simulink model "Model_IPS7"  (R2016a)
settings: Solver=FixedStepAuto  StartTime=0  StopTime=2  FixedStep=1e-5
InitFcn:
  | parametriAM
values from neighbouring files (symbols this model uses):
  filtkonst = 1.3    [parametriAM.m]
  Imrn = 7.4    [parametriAM.m]
  In = 12.7    [parametriAM.m]
  Ismax = In*sqrt(2)    [parametriAM.m]
  J = 0.019    [parametriAM.m]
  Ki_Imr = 1000    [parametriAM.m]
  Ki_tok = 5.0    (= 5)    [parametriAM.m]
  Ki_wr = 1000    [parametriAM.m]
  Kp_Imr = 100    [parametriAM.m]
  Kp_tok = 0.05    [parametriAM.m]
  Kp_wr = 50    [parametriAM.m]
  Lm = 0.0493    [parametriAM.m]
  Lr = 0.05315    [parametriAM.m]
  Ls = 0.05315    [parametriAM.m]
  Lst = sigma*Ls    (= 0.00742111947319)    [parametriAM.m]
  pp = 3    [parametriAM.m]
  Rs = 0.594    [parametriAM.m]
  sigma = 1 - 1/((1+sigmaR)*(1+sigmaS))    (= 0.13962595434)    [parametriAM.m]
  Tr = Lr/Rr    (= 0.0771407837446)    [parametriAM.m]
  Udc = Un*sqrt(2)    [parametriAM.m]
  wb_upper_limit_field_weaking = sqrt((Ls^2+Lst^2)/(2*Lst^2*Ls^2))*Usmax/Ismax    [parametriAM.m]
  wdod = 2000*2*pi/60    (= 209.439510239)    [parametriAM.m]
libraries: simulink x18
(part 1 of 2)
settings Model: Creator=Vaje  LastModifiedBy=Mitja1

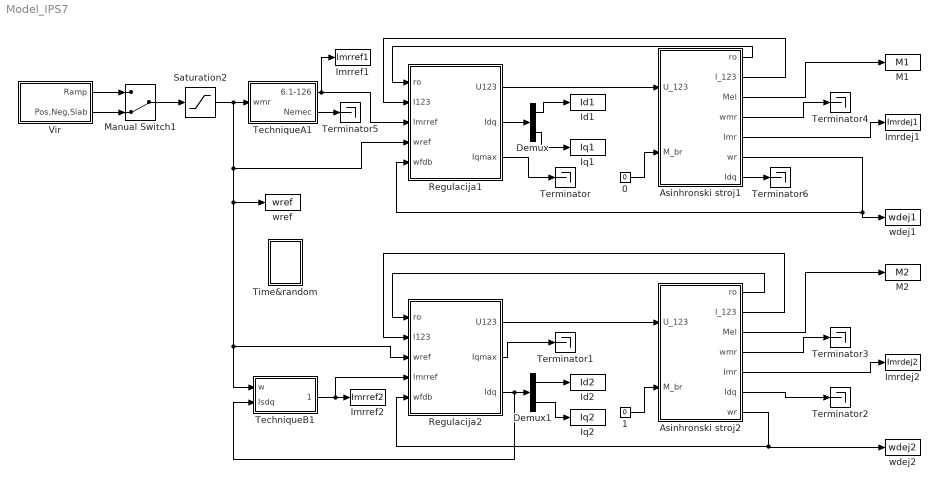
== system Model_IPS7 ==
  0 : Constant  Value=0
  1 : Constant  Value=0
  Asinhronski stroj1 : Subsystem  InitFcn=parametriAM
  Asinhronski stroj2 : Subsystem  InitFcn=parametriAM
  Demux : Demux  Outputs=2
  Demux1 : Demux  Outputs=2
  Id1 : ToWorkspace  VariableName=Id1  SampleTime=-1
      settings: Decimation=3  Save2DSignal=2-D array (concatenate along first dimension)
  Id2 : ToWorkspace  VariableName=Id2  SampleTime=-1
      settings: Decimation=3  Save2DSignal=2-D array (concatenate along first dimension)
  Imrdej1 : ToWorkspace  VariableName=Imrdej1  SampleTime=-1
      settings: Decimation=3  Save2DSignal=2-D array (concatenate along first dimension)
  Imrdej2 : ToWorkspace  VariableName=Imrdej2  SampleTime=-1
      settings: Decimation=3  Save2DSignal=2-D array (concatenate along first dimension)
  Imrref1 : ToWorkspace  VariableName=Imrref1  SampleTime=-1
      settings: Decimation=3  Save2DSignal=2-D array (concatenate along first dimension)
  Imrref2 : ToWorkspace  VariableName=Imrref2  SampleTime=-1
      settings: Decimation=3  Save2DSignal=2-D array (concatenate along first dimension)
  Iq1 : ToWorkspace  VariableName=Iq1  SampleTime=-1
      settings: Decimation=3  Save2DSignal=2-D array (concatenate along first dimension)
  Iq2 : ToWorkspace  VariableName=Iq2  SampleTime=-1
      settings: Decimation=3  Save2DSignal=2-D array (concatenate along first dimension)
  M1 : ToWorkspace  VariableName=M1  SampleTime=-1
      settings: Decimation=3  Save2DSignal=2-D array (concatenate along first dimension)
  M2 : ToWorkspace  VariableName=M2  SampleTime=-1
      settings: Decimation=3  Save2DSignal=2-D array (concatenate along first dimension)
  Manual Switch1 : ManualSwitch  CurrentSetting=0
  Regulacija1 : Subsystem
  Regulacija2 : Subsystem
  Saturation2 : Saturate  UpperLimit=wb_upper_limit_field_weaking  LowerLimit=-wb_upper_limit_field_weaking
  TechniqueA1 : Subsystem
  TechniqueB1 : Subsystem
  Terminator{,1..6} (7 alike) : Terminator
  Time&random : Subsystem
  Vir : Subsystem
  wdej1 : ToWorkspace  VariableName=wdej1  SampleTime=-1
      settings: Decimation=3  Save2DSignal=2-D array (concatenate along first dimension)
  wdej2 : ToWorkspace  VariableName=wdej2  SampleTime=-1
      settings: Decimation=3  Save2DSignal=2-D array (concatenate along first dimension)
  wref : ToWorkspace  VariableName=wref  SampleTime=-1
      settings: Decimation=3  Save2DSignal=2-D array (concatenate along first dimension)
  wires:
  Vir/1(Ramp) -> Manual Switch1/1
  Vir/2(Pos,Neg,Slab) -> Manual Switch1/2
  TechniqueA1/1(6.1-126) -> Regulacija1/3(Imrref), Imrref1/1
  Asinhronski stroj1/1(ro) -> Regulacija1/1(ro)
  Asinhronski stroj1/2(I_123) -> Regulacija1/2(I123)
  Regulacija1/1(U123) -> Asinhronski stroj1/1(U_123)
  Asinhronski stroj1/6(wr) -> Regulacija1/5(wfdb), wdej1/1
  Manual Switch1/1 -> Saturation2/1
  Asinhronski stroj2/1(ro) -> Regulacija2/1(ro)
  Asinhronski stroj2/2(I_123) -> Regulacija2/2(I123)
  Regulacija2/1(U123) -> Asinhronski stroj2/1(U_123)
  Asinhronski stroj2/7(wr) -> Regulacija2/5(wfdb), wdej2/1
  Saturation2/1 -> Regulacija1/4(wref), Regulacija2/3(wref), TechniqueB1/1(w), wref/1, TechniqueA1/1(wmr)
  Regulacija2/3(Idq) -> TechniqueB1/2(Isdq), Demux1/1
  TechniqueB1/1(6.1-135) -> Regulacija2/4(Imrref), Imrref2/1
  Asinhronski stroj1/5(Imr) -> Imrdej1/1
  Asinhronski stroj2/5(Imr) -> Imrdej2/1
  Asinhronski stroj1/3(Mel) -> M1/1
  Asinhronski stroj2/3(Mel) -> M2/1
  Demux/2 -> Iq1/1
  Demux/1 -> Id1/1
  Demux1/1 -> Id2/1
  Demux1/2 -> Iq2/1
  Regulacija1/2(Idq) -> Demux/1
  Regulacija1/3(Iqmax) -> Terminator/1
  Regulacija2/2(Iqmax) -> Terminator1/1
  Asinhronski stroj2/6(Idq) -> Terminator2/1
  Asinhronski stroj2/4(wmr) -> Terminator3/1
  Asinhronski stroj1/4(wmr) -> Terminator4/1
  TechniqueA1/2(Nemec) -> Terminator5/1
  0/1 -> Asinhronski stroj1/2(M_br)
  1/1 -> Asinhronski stroj2/2(M_br)
  Asinhronski stroj1/7(Idq) -> Terminator6/1

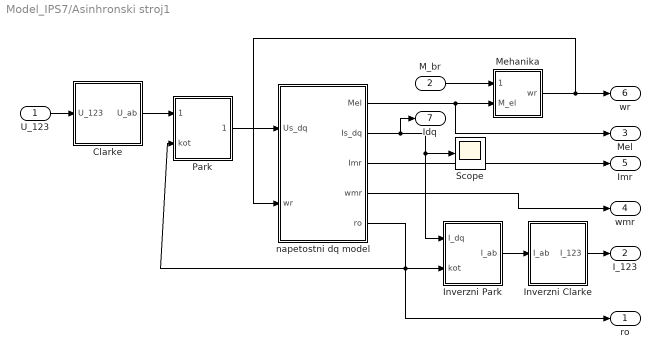
== system Model_IPS7/Asinhronski stroj1 ==
  U_123 : Inport
  M_br : Inport  Port=2
  Clarke : Subsystem
  Inverzni Clarke : Subsystem
  Inverzni Park : Subsystem
  Mehanika : Subsystem
  Park : Subsystem
  Scope : Scope
  napetostni dq model : Subsystem
  ro : Outport
  I_123 : Outport  Port=2
  Mel : Outport  Port=3
  wmr : Outport  Port=4
  Imr : Outport  Port=5
  wr : Outport  Port=6
  Idq : Outport  Port=7
  wires:
  Inverzni Park/1(I_ab) -> Inverzni Clarke/1(I_ab)
  Clarke/1(U_ab) -> Park/1(U_ab)
  Mehanika/1(wr) -> napetostni dq model/2(wr), wr/1
  M_br/1 -> Mehanika/1(M_br)
  napetostni dq model/1(Mel) -> Mel/1, Mehanika/2(M_el)
  Inverzni Clarke/1(I_123) -> I_123/1
  napetostni dq model/4(wmr) -> wmr/1
  napetostni dq model/3(Imr) -> Imr/1
  U_123/1 -> Clarke/1(U_123)
  napetostni dq model/2(Is_dq) -> Idq/1, Scope/1, Inverzni Park/1(I_dq)
  napetostni dq model/5(ro) -> ro/1, Park/2(kot), Inverzni Park/2(kot)
  Park/1(U_dq) -> napetostni dq model/1(Us_dq)

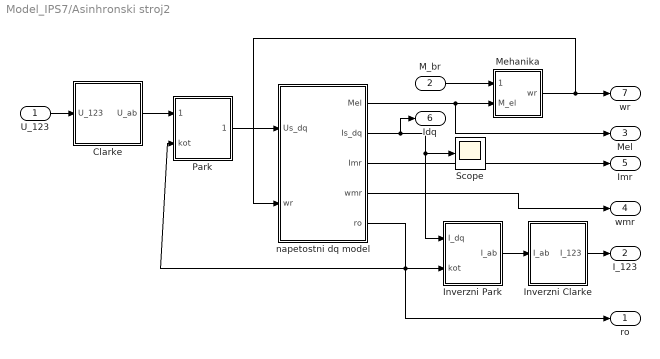
== system Model_IPS7/Asinhronski stroj2 ==
  U_123 : Inport
  M_br : Inport  Port=2
  Clarke : Subsystem
  Inverzni Clarke : Subsystem
  Inverzni Park : Subsystem
  Mehanika : Subsystem
  Park : Subsystem
  Scope : Scope
  napetostni dq model : Subsystem
  ro : Outport
  I_123 : Outport  Port=2
  Mel : Outport  Port=3
  wmr : Outport  Port=4
  Imr : Outport  Port=5
  Idq : Outport  Port=6
  wr : Outport  Port=7
  wires:
  Inverzni Park/1(I_ab) -> Inverzni Clarke/1(I_ab)
  Clarke/1(U_ab) -> Park/1(U_ab)
  Mehanika/1(wr) -> napetostni dq model/2(wr), wr/1
  M_br/1 -> Mehanika/1(M_br)
  napetostni dq model/1(Mel) -> Mel/1, Mehanika/2(M_el)
  Inverzni Clarke/1(I_123) -> I_123/1
  napetostni dq model/4(wmr) -> wmr/1
  napetostni dq model/3(Imr) -> Imr/1
  U_123/1 -> Clarke/1(U_123)
  napetostni dq model/2(Is_dq) -> Idq/1, Scope/1, Inverzni Park/1(I_dq)
  napetostni dq model/5(ro) -> ro/1, Park/2(kot), Inverzni Park/2(kot)
  Park/1(U_dq) -> napetostni dq model/1(Us_dq)

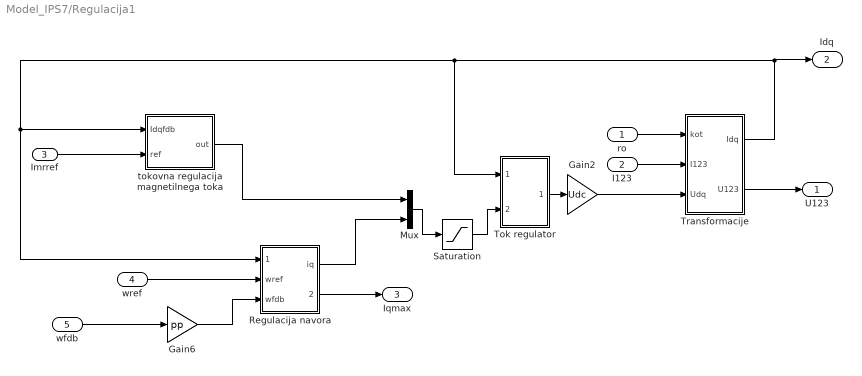
== system Model_IPS7/Regulacija1 ==
  ro : Inport
  I123 : Inport  Port=2
  Imrref : Inport  Port=3
  wref : Inport  Port=4
  wfdb : Inport  Port=5
  Gain2 : Gain  Gain=Udc
  Gain6 : Gain  Gain=pp
  Mux : Mux  Inputs=2
  Regulacija navora : Subsystem
  Saturation : Saturate  UpperLimit=Ismax  LowerLimit=-Ismax
  Tok regulator : Subsystem
  Transformacije : Subsystem
  tokovna regulacija magnetilnega toka : Subsystem
  U123 : Outport
  Idq : Outport  Port=2
  Iqmax : Outport  Port=3
  wires:
  Imrref/1 -> tokovna regulacija magnetilnega toka/2(ref)
  wref/1 -> Regulacija navora/2(wref)
  Transformacije/1(Idq) -> Tok regulator/1(Idqdej), Regulacija navora/1(Idqdej), tokovna regulacija magnetilnega toka/1(Idqfdb), Idq/1
  ro/1 -> Transformacije/1(kot)
  I123/1 -> Transformacije/2(I123)
  Gain2/1 -> Transformacije/3(Udq)
  wfdb/1 -> Gain6/1
  tokovna regulacija magnetilnega toka/1(out) -> Mux/1
  Mux/1 -> Saturation/1
  Tok regulator/1(Udq) -> Gain2/1
  Regulacija navora/1(iq) -> Mux/2
  Transformacije/2(U123) -> U123/1
  Regulacija navora/2(Iqmax) -> Iqmax/1
  Gain6/1 -> Regulacija navora/3(wfdb)
  Saturation/1 -> Tok regulator/2(Idqref)

== system Model_IPS7/Regulacija2 ==
  ro : Inport
  I123 : Inport  Port=2
  wref : Inport  Port=3
  Imrref : Inport  Port=4
  wfdb : Inport  Port=5
  Gain2 : Gain  Gain=Udc
  Gain6 : Gain  Gain=pp
  Mux : Mux  Inputs=2
  Regulacija navora : Subsystem
  Tok regulator : Subsystem
  Transformacije : Subsystem
  tokovna regulacija magnetilnega toka : Subsystem
  U123 : Outport
  Iqmax : Outport  Port=2
  Idq : Outport  Port=3
  wires:
  Imrref/1 -> tokovna regulacija magnetilnega toka/2(ref)
  wref/1 -> Regulacija navora/2(wref)
  Transformacije/1(Idq) -> Tok regulator/1(Idqdej), Regulacija navora/1(Idqdej), tokovna regulacija magnetilnega toka/1(Idqfdb), Idq/1
  ro/1 -> Transformacije/1(kot)
  I123/1 -> Transformacije/2(I123)
  Gain2/1 -> Transformacije/3(Udq)
  wfdb/1 -> Gain6/1
  tokovna regulacija magnetilnega toka/1(out) -> Mux/1
  Mux/1 -> Tok regulator/2(Idqref)
  Tok regulator/1(Udq) -> Gain2/1
  Regulacija navora/1(iq) -> Mux/2
  Transformacije/2(U123) -> U123/1
  Regulacija navora/2(Iqmax) -> Iqmax/1
  Gain6/1 -> Regulacija navora/3(wfdb)

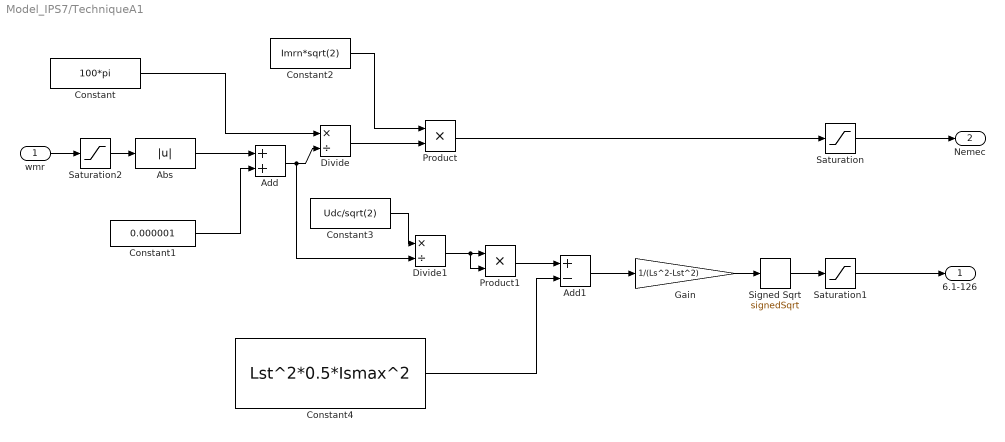
== system Model_IPS7/TechniqueA1 ==
  wmr : Inport
  Abs : Abs
  Add : Sum
  Add1 : Sum  Inputs=+-
  Constant : Constant  Value=100*pi
  Constant1 : Constant  Value=0.000001
  Constant2 : Constant  Value=Imrn*sqrt(2)
  Constant3 : Constant  Value=Udc/sqrt(2)
  Constant4 : Constant  Value=Lst^2*0.5*Ismax^2
  Divide : Product  Inputs=*/
  Divide1 : Product  Inputs=*/
  Gain : Gain  Gain=1/(Ls^2-Lst^2)
  Product : Product
  Product1 : Product
  Saturation : Saturate  UpperLimit=+Imrn*sqrt(2)  LowerLimit=0
  Saturation1 : Saturate  UpperLimit=+Imrn*sqrt(2)  LowerLimit=-Imrn*sqrt(2)
  Saturation2 : Saturate  UpperLimit=wb_upper_limit_field_weaking  LowerLimit=-wb_upper_limit_field_weaking
  Signed Sqrt : Sqrt  Operator=signedSqrt  SaturateOnIntegerOverflow=on
  6.1-126 : Outport
  Nemec : Outport  Port=2
  wires:
  Constant2/1 -> Product/1
  Divide/1 -> Product/2
  Product/1 -> Saturation/1
  Constant/1 -> Divide/1
  Add/1 -> Divide1/2, Divide/2
  Abs/1 -> Add/1
  Constant1/1 -> Add/2
  Saturation/1 -> Nemec/1
  Constant3/1 -> Divide1/1
  Divide1/1 -> Product1/2, Product1/1
  Product1/1 -> Add1/1
  Constant4/1 -> Add1/2
  Saturation1/1 -> 6.1-126/1
  Add1/1 -> Gain/1
  Gain/1 -> Signed Sqrt/1
  Signed Sqrt/1 -> Saturation1/1
  wmr/1 -> Saturation2/1
  Saturation2/1 -> Abs/1

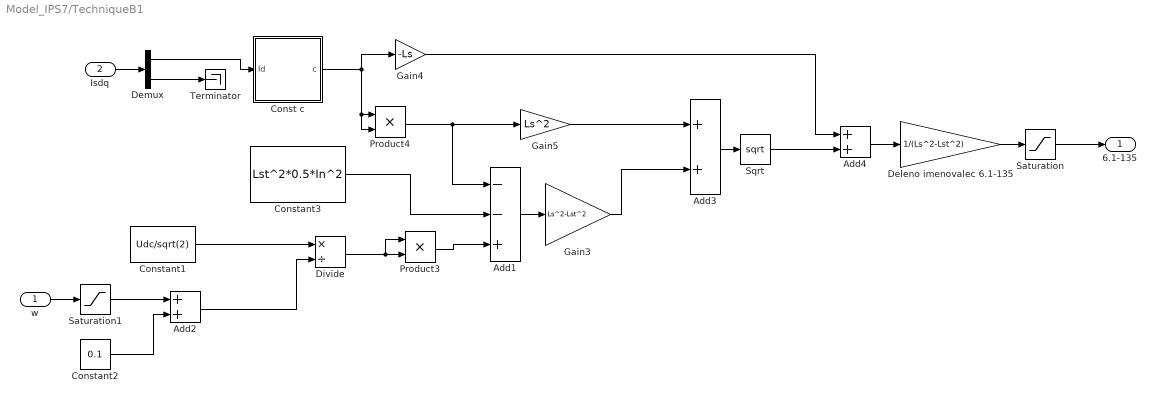
== system Model_IPS7/TechniqueB1 ==
  w : Inport
  Isdq : Inport  Port=2
  Add1 : Sum  Inputs=--+
  Add2 : Sum
  Add3 : Sum
  Add4 : Sum
  Const c : Subsystem
  Constant1 : Constant  Value=Udc/sqrt(2)
  Constant2 : Constant  Value=0.1
  Constant3 : Constant  Value=Lst^2*0.5*In^2
  Deleno imenovalec 6.1-135 : Gain  Gain=1/(Ls^2-Lst^2)
  Demux : Demux  Outputs=2
  Divide : Product  Inputs=*/
  Gain3 : Gain  Gain=Ls^2-Lst^2
  Gain4 : Gain  Gain=-Ls
  Gain5 : Gain  Gain=Ls^2
  Product3 : Product
  Product4 : Product
  Saturation : Saturate  UpperLimit=+Imrn*sqrt(2)  LowerLimit=-Imrn*sqrt(2)
  Saturation1 : Saturate  UpperLimit=wb_upper_limit_field_weaking  LowerLimit=-wb_upper_limit_field_weaking
  Sqrt : Sqrt  SaturateOnIntegerOverflow=on
  Terminator : Terminator
  6.1-135 : Outport
  wires:
  Constant1/1 -> Divide/1
  w/1 -> Saturation1/1
  Constant2/1 -> Add2/2
  Demux/1 -> Const c/1(Id)
  Demux/2 -> Terminator/1
  Saturation/1 -> 6.1-135/1
  Const c/1(c) -> Gain4/1, Product4/2, Product4/1
  Product4/1 -> Add1/1, Gain5/1
  Gain5/1 -> Add3/1
  Gain4/1 -> Add4/1
  Add4/1 -> Deleno imenovalec 6.1-135/1
  Deleno imenovalec 6.1-135/1 -> Saturation/1
  Add1/1 -> Gain3/1
  Constant3/1 -> Add1/2
  Add2/1 -> Divide/2
  Divide/1 -> Product3/1, Product3/2
  Product3/1 -> Add1/3
  Sqrt/1 -> Add4/2
  Add3/1 -> Sqrt/1
  Gain3/1 -> Add3/2
  Saturation1/1 -> Add2/1
  Isdq/1 -> Demux/1

== system Model_IPS7/Time&random ==
  99% max navora : Subsystem  Commented=on
  Mux1 : Mux  Commented=on  Inputs=2
  Ramp : simulink/Sources/Ramp  slope=1  start=0  X0=0
  To Workspace3 : ToWorkspace  VariableName=time  SampleTime=-1
      settings: Decimation=3  Save2DSignal=2-D array (concatenate along first dimension)
  wires:
  Ramp/1 -> To Workspace3/1

== system Model_IPS7/Vir ==
  Add1 : Sum
  Rampa : simulink/Sources/Ramp  slope=500*2*pi/60  start=0.5  X0=0
  Step : Step  Time=0.1  After=2000*2*pi/60  SampleTime=0
  Step1 : Step  Time=0.7  After=2000*pi/30  SampleTime=0
  Step2 : Step  Commented=on  Time=2  After=2000*2*pi/60  SampleTime=0
  Step3 : Step  Commented=on  Time=3  After=2000*2*pi/60  SampleTime=0
  Step4 : Step  Commented=on  Time=8  After=wdod  SampleTime=0
  Step5 : Step  Commented=on  Time=9  After=wdod  SampleTime=0
  Ramp : Outport
  Pos,Neg,Slab : Outport  Port=2
  wires:
  Add1/1 -> Pos,Neg,Slab/1
  Step/1 -> Add1/1
  Rampa/1 -> Ramp/1
  Step1/1 -> Add1/2

== system Model_IPS7/Asinhronski stroj1/Clarke ==
  U_123 : Inport
  ABC_ab1 : Subsystem
  Demux : Demux  Outputs=3
  Mux : Mux  Inputs=2
  U_ab : Outport
  wires:
  Mux/1 -> U_ab/1
  ABC_ab1/2(beta) -> Mux/2
  ABC_ab1/1(alfa) -> Mux/1
  Demux/3 -> ABC_ab1/3(C)
  Demux/2 -> ABC_ab1/2(B)
  Demux/1 -> ABC_ab1/1(A)
  U_123/1 -> Demux/1

== system Model_IPS7/Asinhronski stroj1/Inverzni Clarke ==
  I_ab : Inport
  Demux : Demux  Outputs=2
  Mux : Mux  Inputs=3
  ab_ABC : Subsystem
  I_123 : Outport
  wires:
  ab_ABC/3(C) -> Mux/3
  ab_ABC/2(B) -> Mux/2
  ab_ABC/1(A) -> Mux/1
  Demux/2 -> ab_ABC/2(beta)
  Demux/1 -> ab_ABC/1(alfa)
  I_ab/1 -> Demux/1
  Mux/1 -> I_123/1

== system Model_IPS7/Asinhronski stroj1/Inverzni Park ==
  I_dq : Inport
  kot : Inport  Port=2
  Demux : Demux  Outputs=2
  Mux : Mux  Inputs=2
  "Sum1 " : Sum  Inputs=+-  SaturateOnIntegerOverflow=on  InputSameDT=on  OutDataTypeStr=Inherit: Same as first input
  Sum2 : Sum  SaturateOnIntegerOverflow=on  InputSameDT=on  OutDataTypeStr=Inherit: Same as first input
  cos : Fcn  Expr=cos(u)
  sin : Fcn  Expr=sin(u)
  x_d*cos : Product  SaturateOnIntegerOverflow=on  RndMeth=Zero  InputSameDT=on  OutDataTypeStr=Inherit: Same as first input
  x_d*sin : Product  SaturateOnIntegerOverflow=on  RndMeth=Zero  InputSameDT=on  OutDataTypeStr=Inherit: Same as first input
  x_q*cos : Product  SaturateOnIntegerOverflow=on  RndMeth=Zero  InputSameDT=on  OutDataTypeStr=Inherit: Same as first input
  "x_q*sin " : Product  SaturateOnIntegerOverflow=on  RndMeth=Zero  InputSameDT=on  OutDataTypeStr=Inherit: Same as first input
  I_ab : Outport
  wires:
  Mux/1 -> I_ab/1
  I_dq/1 -> Demux/1
  Demux/1 -> x_d*sin/1, x_d*cos/1
  Demux/2 -> "x_q*sin "/1, x_q*cos/1
  cos/1 -> x_q*cos/2, x_d*cos/2
  sin/1 -> "x_q*sin "/2, x_d*sin/2
  x_d*cos/1 -> "Sum1 "/1
  "x_q*sin "/1 -> "Sum1 "/2
  x_q*cos/1 -> Sum2/2
  x_d*sin/1 -> Sum2/1
  "Sum1 "/1 -> Mux/1
  Sum2/1 -> Mux/2
  kot/1 -> cos/1, sin/1

== system Model_IPS7/Asinhronski stroj1/Mehanika ==
  M_br : Inport
  M_el : Inport  Port=2
  Sum : Sum  Inputs=+-
  eq 2.19 : Subsystem
  wr : Outport
  wires:
  M_br/1 -> Sum/2
  Sum/1 -> eq 2.19/1(M)
  M_el/1 -> Sum/1
  eq 2.19/1(wr) -> wr/1

== system Model_IPS7/Asinhronski stroj1/Park ==
  U_ab : Inport
  kot : Inport  Port=2
  Demux : Demux  Outputs=2
  Mux : Mux  Inputs=2
  "Sum1 " : Sum  SaturateOnIntegerOverflow=on  InputSameDT=on  OutDataTypeStr=Inherit: Same as first input
  Sum2 : Sum  Inputs=-+  SaturateOnIntegerOverflow=on  InputSameDT=on  OutDataTypeStr=Inherit: Same as first input
  cos : Fcn  Expr=cos(u)
  sin : Fcn  Expr=sin(u)
  x_a*cos : Product  SaturateOnIntegerOverflow=on  RndMeth=Zero  InputSameDT=on  OutDataTypeStr=Inherit: Same as first input
  x_a*sin : Product  SaturateOnIntegerOverflow=on  RndMeth=Zero  InputSameDT=on  OutDataTypeStr=Inherit: Same as first input
  x_b*cos : Product  SaturateOnIntegerOverflow=on  RndMeth=Zero  InputSameDT=on  OutDataTypeStr=Inherit: Same as first input
  "x_b*sin " : Product  SaturateOnIntegerOverflow=on  RndMeth=Zero  InputSameDT=on  OutDataTypeStr=Inherit: Same as first input
  U_dq : Outport
  wires:
  Mux/1 -> U_dq/1
  U_ab/1 -> Demux/1
  Demux/1 -> x_a*sin/1, x_a*cos/1
  Demux/2 -> "x_b*sin "/1, x_b*cos/1
  cos/1 -> x_b*cos/2, x_a*cos/2
  sin/1 -> "x_b*sin "/2, x_a*sin/2
  x_a*cos/1 -> "Sum1 "/1
  "x_b*sin "/1 -> "Sum1 "/2
  x_b*cos/1 -> Sum2/2
  x_a*sin/1 -> Sum2/1
  "Sum1 "/1 -> Mux/1
  Sum2/1 -> Mux/2
  kot/1 -> cos/1, sin/1

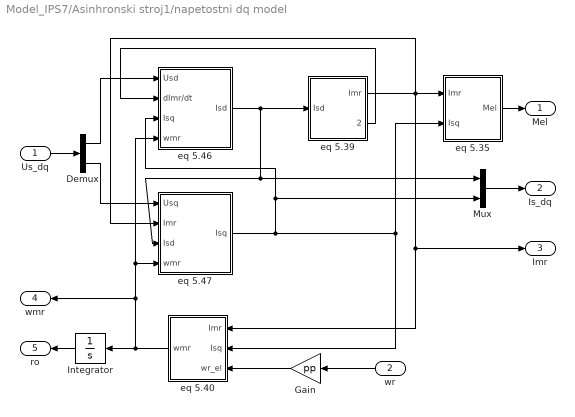
== system Model_IPS7/Asinhronski stroj1/napetostni dq model ==
  Us_dq : Inport
  wr : Inport  Port=2
  Demux : Demux  Outputs=2
  Gain : Gain  Gain=pp
  Integrator : Integrator
  Mux : Mux  Inputs=2
  eq 5.35 : Subsystem
  eq 5.39 : Subsystem
  eq 5.40 : Subsystem
  eq 5.46 : Subsystem
  eq 5.47 : Subsystem
  Mel : Outport
  Is_dq : Outport  Port=2
  Imr : Outport  Port=3
  wmr : Outport  Port=4
  ro : Outport  Port=5
  wires:
  Gain/1 -> eq 5.40/3(wr_el)
  Mux/1 -> Is_dq/1
  Demux/2 -> eq 5.47/1(Usq)
  Demux/1 -> eq 5.46/1(Usd)
  Us_dq/1 -> Demux/1
  wr/1 -> Gain/1
  Integrator/1 -> ro/1
  eq 5.35/1(Mel) -> Mel/1
  eq 5.40/1(wmr) -> Integrator/1, wmr/1, eq 5.46/4(wmr), eq 5.47/4(wmr)
  eq 5.47/1(Isq) -> Mux/2, eq 5.46/3(Isq), eq 5.40/2(Isq), eq 5.35/2(Isq)
  eq 5.39/1(Imr) -> eq 5.47/2(Imr), Imr/1, eq 5.40/1(Imr), eq 5.35/1(Imr)
  eq 5.39/2(dImr/dt) -> eq 5.46/2(dImr/dt)
  eq 5.46/1(Isd) -> Mux/1, eq 5.47/3(Isd), eq 5.39/1(Isd)

== system Model_IPS7/Asinhronski stroj2/Clarke ==
  U_123 : Inport
  ABC_ab1 : Subsystem
  Demux : Demux  Outputs=3
  Mux : Mux  Inputs=2
  U_ab : Outport
  wires:
  Mux/1 -> U_ab/1
  ABC_ab1/2(beta) -> Mux/2
  ABC_ab1/1(alfa) -> Mux/1
  Demux/3 -> ABC_ab1/3(C)
  Demux/2 -> ABC_ab1/2(B)
  Demux/1 -> ABC_ab1/1(A)
  U_123/1 -> Demux/1

== system Model_IPS7/Asinhronski stroj2/Inverzni Clarke ==
  I_ab : Inport
  Demux : Demux  Outputs=2
  Mux : Mux  Inputs=3
  ab_ABC : Subsystem
  I_123 : Outport
  wires:
  ab_ABC/3(C) -> Mux/3
  ab_ABC/2(B) -> Mux/2
  ab_ABC/1(A) -> Mux/1
  Demux/2 -> ab_ABC/2(beta)
  Demux/1 -> ab_ABC/1(alfa)
  I_ab/1 -> Demux/1
  Mux/1 -> I_123/1

== system Model_IPS7/Asinhronski stroj2/Inverzni Park ==
  I_dq : Inport
  kot : Inport  Port=2
  Demux : Demux  Outputs=2
  Mux : Mux  Inputs=2
  "Sum1 " : Sum  Inputs=+-  SaturateOnIntegerOverflow=on  InputSameDT=on  OutDataTypeStr=Inherit: Same as first input
  Sum2 : Sum  SaturateOnIntegerOverflow=on  InputSameDT=on  OutDataTypeStr=Inherit: Same as first input
  cos : Fcn  Expr=cos(u)
  sin : Fcn  Expr=sin(u)
  x_d*cos : Product  SaturateOnIntegerOverflow=on  RndMeth=Zero  InputSameDT=on  OutDataTypeStr=Inherit: Same as first input
  x_d*sin : Product  SaturateOnIntegerOverflow=on  RndMeth=Zero  InputSameDT=on  OutDataTypeStr=Inherit: Same as first input
  x_q*cos : Product  SaturateOnIntegerOverflow=on  RndMeth=Zero  InputSameDT=on  OutDataTypeStr=Inherit: Same as first input
  "x_q*sin " : Product  SaturateOnIntegerOverflow=on  RndMeth=Zero  InputSameDT=on  OutDataTypeStr=Inherit: Same as first input
  I_ab : Outport
  wires:
  Mux/1 -> I_ab/1
  I_dq/1 -> Demux/1
  Demux/1 -> x_d*sin/1, x_d*cos/1
  Demux/2 -> "x_q*sin "/1, x_q*cos/1
  cos/1 -> x_q*cos/2, x_d*cos/2
  sin/1 -> "x_q*sin "/2, x_d*sin/2
  x_d*cos/1 -> "Sum1 "/1
  "x_q*sin "/1 -> "Sum1 "/2
  x_q*cos/1 -> Sum2/2
  x_d*sin/1 -> Sum2/1
  "Sum1 "/1 -> Mux/1
  Sum2/1 -> Mux/2
  kot/1 -> cos/1, sin/1

== system Model_IPS7/Asinhronski stroj2/Mehanika ==
  M_br : Inport
  M_el : Inport  Port=2
  Sum : Sum  Inputs=+-
  eq 2.19 : Subsystem
  wr : Outport
  wires:
  M_br/1 -> Sum/2
  Sum/1 -> eq 2.19/1(M)
  M_el/1 -> Sum/1
  eq 2.19/1(wr) -> wr/1

== system Model_IPS7/Asinhronski stroj2/Park ==
  U_ab : Inport
  kot : Inport  Port=2
  Demux : Demux  Outputs=2
  Mux : Mux  Inputs=2
  "Sum1 " : Sum  SaturateOnIntegerOverflow=on  InputSameDT=on  OutDataTypeStr=Inherit: Same as first input
  Sum2 : Sum  Inputs=-+  SaturateOnIntegerOverflow=on  InputSameDT=on  OutDataTypeStr=Inherit: Same as first input
  cos : Fcn  Expr=cos(u)
  sin : Fcn  Expr=sin(u)
  x_a*cos : Product  SaturateOnIntegerOverflow=on  RndMeth=Zero  InputSameDT=on  OutDataTypeStr=Inherit: Same as first input
  x_a*sin : Product  SaturateOnIntegerOverflow=on  RndMeth=Zero  InputSameDT=on  OutDataTypeStr=Inherit: Same as first input
  x_b*cos : Product  SaturateOnIntegerOverflow=on  RndMeth=Zero  InputSameDT=on  OutDataTypeStr=Inherit: Same as first input
  "x_b*sin " : Product  SaturateOnIntegerOverflow=on  RndMeth=Zero  InputSameDT=on  OutDataTypeStr=Inherit: Same as first input
  U_dq : Outport
  wires:
  Mux/1 -> U_dq/1
  U_ab/1 -> Demux/1
  Demux/1 -> x_a*sin/1, x_a*cos/1
  Demux/2 -> "x_b*sin "/1, x_b*cos/1
  cos/1 -> x_b*cos/2, x_a*cos/2
  sin/1 -> "x_b*sin "/2, x_a*sin/2
  x_a*cos/1 -> "Sum1 "/1
  "x_b*sin "/1 -> "Sum1 "/2
  x_b*cos/1 -> Sum2/2
  x_a*sin/1 -> Sum2/1
  "Sum1 "/1 -> Mux/1
  Sum2/1 -> Mux/2
  kot/1 -> cos/1, sin/1

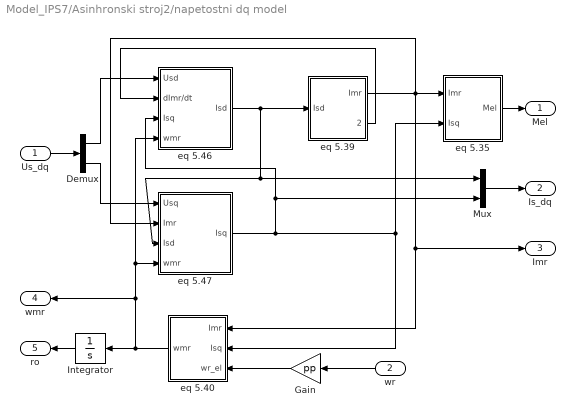
== system Model_IPS7/Asinhronski stroj2/napetostni dq model ==
  Us_dq : Inport
  wr : Inport  Port=2
  Demux : Demux  Outputs=2
  Gain : Gain  Gain=pp
  Integrator : Integrator
  Mux : Mux  Inputs=2
  eq 5.35 : Subsystem
  eq 5.39 : Subsystem
  eq 5.40 : Subsystem
  eq 5.46 : Subsystem
  eq 5.47 : Subsystem
  Mel : Outport
  Is_dq : Outport  Port=2
  Imr : Outport  Port=3
  wmr : Outport  Port=4
  ro : Outport  Port=5
  wires:
  Gain/1 -> eq 5.40/3(wr_el)
  Mux/1 -> Is_dq/1
  Demux/2 -> eq 5.47/1(Usq)
  Demux/1 -> eq 5.46/1(Usd)
  Us_dq/1 -> Demux/1
  wr/1 -> Gain/1
  Integrator/1 -> ro/1
  eq 5.35/1(Mel) -> Mel/1
  eq 5.40/1(wmr) -> Integrator/1, wmr/1, eq 5.46/4(wmr), eq 5.47/4(wmr)
  eq 5.47/1(Isq) -> Mux/2, eq 5.46/3(Isq), eq 5.40/2(Isq), eq 5.35/2(Isq)
  eq 5.39/1(Imr) -> eq 5.47/2(Imr), Imr/1, eq 5.40/1(Imr), eq 5.35/1(Imr)
  eq 5.39/2(dImr/dt) -> eq 5.46/2(dImr/dt)
  eq 5.46/1(Isd) -> Mux/1, eq 5.47/3(Isd), eq 5.39/1(Isd)

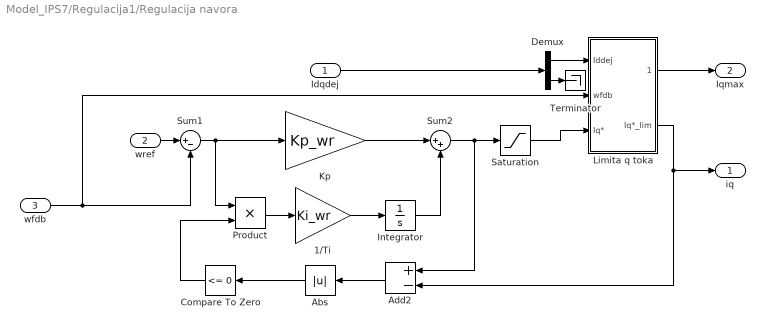
== system Model_IPS7/Regulacija1/Regulacija navora ==
  Idqdej : Inport
  wref : Inport  Port=2
  wfdb : Inport  Port=3
  1/Ti : Gain  Gain=Ki_wr  SaturateOnIntegerOverflow=on  OutDataTypeStr=Inherit: Same as input  ParamDataTypeStr=Inherit: Same as input
  Abs : Abs
  Add2 : Sum  Inputs=+-
  Compare To Zero : simulink/Logic and Bit Operations/Compare To Zero  relop=<=  OutDataTypeStr=boolean
  Demux : Demux  Outputs=2
  Integrator : Integrator
  Kp : Gain  Gain=Kp_wr  SaturateOnIntegerOverflow=on  OutDataTypeStr=Inherit: Same as input  ParamDataTypeStr=Inherit: Same as input
  Limita q toka : Subsystem
  Product : Product
  Saturation : Saturate  UpperLimit=Ismax  LowerLimit=-Ismax
  Sum1 : Sum  Inputs=|+-
  Sum2 : Sum  Inputs=|++
  Terminator : Terminator
  iq : Outport
  Iqmax : Outport  Port=2
  wires:
  1/Ti/1 -> Integrator/1
  Sum1/1 -> Product/1, Kp/1
  Integrator/1 -> Sum2/2
  Add2/1 -> Abs/1
  Abs/1 -> Compare To Zero/1
  Kp/1 -> Sum2/1
  Compare To Zero/1 -> Product/2
  Product/1 -> 1/Ti/1
  wref/1 -> Sum1/1
  wfdb/1 -> Sum1/2, Limita q toka/2(wfdb)
  Sum2/1 -> Saturation/1, Add2/1
  Limita q toka/2(Iq*_lim) -> iq/1, Add2/2
  Idqdej/1 -> Demux/1
  Limita q toka/1(Iqmaxlim) -> Iqmax/1
  Demux/1 -> Limita q toka/1(Iddej)
  Demux/2 -> Terminator/1
  Saturation/1 -> Limita q toka/3(Iq*)

== system Model_IPS7/Regulacija1/Tok regulator ==
  Idqdej : Inport
  Idqref : Inport  Port=2
  Demux : Demux  Outputs=2
  Demux1 : Demux  Outputs=2
  Dregulator : Subsystem
  Limita Uq : Subsystem
  Mux : Mux  Inputs=2
  Qregulator : Subsystem
  Udq : Outport
  wires:
  Idqref/1 -> Demux1/1
  Mux/1 -> Udq/1
  Idqdej/1 -> Demux/1
  Limita Uq/1(Uq_lim) -> Qregulator/3(Uqlim), Mux/2
  Dregulator/1(Ud*(-1:1)) -> Mux/1, Limita Uq/1(Ud)
  Demux1/1 -> Dregulator/1(Id*)
  Demux/1 -> Dregulator/2(Iddej)
  Demux1/2 -> Qregulator/2(Iq*)
  Demux/2 -> Qregulator/1(Iqdej)
  Qregulator/1(Uq*(-1:1)) -> Limita Uq/2(Uq)

== system Model_IPS7/Regulacija1/Transformacije ==
  kot : Inport
  I123 : Inport  Port=2
  Udq : Inport  Port=3
  Clarke : Subsystem
  Inverzni Clarke : Subsystem
  Inverzni Park : Subsystem
  Park : Subsystem
  Idq : Outport
  U123 : Outport  Port=2
  wires:
  Inverzni Clarke/1(U_123) -> U123/1
  Park/1(I_dq) -> Idq/1
  kot/1 -> Inverzni Park/1(kot), Park/2(kot)
  Clarke/1(I_ab) -> Park/1(I_ab)
  Inverzni Park/1(U_ab) -> Inverzni Clarke/1(U_ab)
  Udq/1 -> Inverzni Park/2(U_dq)
  I123/1 -> Clarke/1(I_123)

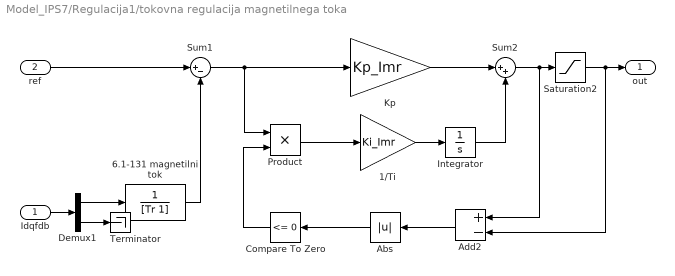
== system Model_IPS7/Regulacija1/tokovna regulacija magnetilnega toka ==
  Idqfdb : Inport
  ref : Inport  Port=2
  1/Ti : Gain  Gain=Ki_Imr  SaturateOnIntegerOverflow=on  OutDataTypeStr=Inherit: Same as input  ParamDataTypeStr=Inherit: Same as input
  6.1-131 magnetilni tok : TransferFcn  Denominator=[Tr 1]
  Abs : Abs
  Add2 : Sum  Inputs=+-
  Compare To Zero : simulink/Logic and Bit Operations/Compare To Zero  relop=<=  OutDataTypeStr=boolean
  Demux1 : Demux  Outputs=2
  Integrator : Integrator
  Kp : Gain  Gain=Kp_Imr  SaturateOnIntegerOverflow=on  OutDataTypeStr=Inherit: Same as input  ParamDataTypeStr=Inherit: Same as input
  Product : Product
  Saturation2 : Saturate  UpperLimit=Ismax  LowerLimit=-Ismax
  Sum1 : Sum  Inputs=|+-
  Sum2 : Sum  Inputs=|++
  Terminator : Terminator
  out : Outport
  wires:
  Product/1 -> 1/Ti/1
  Compare To Zero/1 -> Product/2
  Abs/1 -> Compare To Zero/1
  Add2/1 -> Abs/1
  Integrator/1 -> Sum2/2
  ref/1 -> Sum1/1
  Sum1/1 -> Kp/1, Product/1
  1/Ti/1 -> Integrator/1
  Kp/1 -> Sum2/1
  Demux1/1 -> 6.1-131 magnetilni tok/1
  6.1-131 magnetilni tok/1 -> Sum1/2
  Idqfdb/1 -> Demux1/1
  Sum2/1 -> Add2/1, Saturation2/1
  Saturation2/1 -> Add2/2, out/1
  Demux1/2 -> Terminator/1

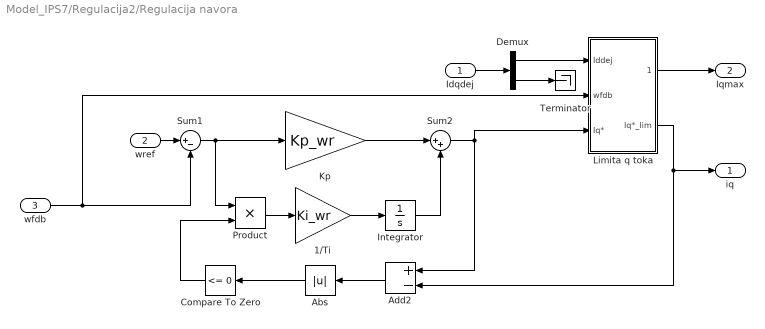
== system Model_IPS7/Regulacija2/Regulacija navora ==
  Idqdej : Inport
  wref : Inport  Port=2
  wfdb : Inport  Port=3
  1/Ti : Gain  Gain=Ki_wr  SaturateOnIntegerOverflow=on  OutDataTypeStr=Inherit: Same as input  ParamDataTypeStr=Inherit: Same as input
  Abs : Abs
  Add2 : Sum  Inputs=+-
  Compare To Zero : simulink/Logic and Bit Operations/Compare To Zero  relop=<=  OutDataTypeStr=boolean
  Demux : Demux  Outputs=2
  Integrator : Integrator
  Kp : Gain  Gain=Kp_wr  SaturateOnIntegerOverflow=on  OutDataTypeStr=Inherit: Same as input  ParamDataTypeStr=Inherit: Same as input
  Limita q toka : Subsystem
  Product : Product
  Sum1 : Sum  Inputs=|+-
  Sum2 : Sum  Inputs=|++
  Terminator : Terminator
  iq : Outport
  Iqmax : Outport  Port=2
  wires:
  1/Ti/1 -> Integrator/1
  Sum1/1 -> Product/1, Kp/1
  Integrator/1 -> Sum2/2
  Add2/1 -> Abs/1
  Abs/1 -> Compare To Zero/1
  Kp/1 -> Sum2/1
  Compare To Zero/1 -> Product/2
  Product/1 -> 1/Ti/1
  wref/1 -> Sum1/1
  wfdb/1 -> Sum1/2, Limita q toka/2(wfdb)
  Sum2/1 -> Add2/1, Limita q toka/3(Iq*)
  Limita q toka/2(Iq*_lim) -> iq/1, Add2/2
  Idqdej/1 -> Demux/1
  Limita q toka/1(Iqmaxlim) -> Iqmax/1
  Demux/1 -> Limita q toka/1(Iddej)
  Demux/2 -> Terminator/1

== system Model_IPS7/Regulacija2/Tok regulator ==
  Idqdej : Inport
  Idqref : Inport  Port=2
  Demux : Demux  Outputs=2
  Demux1 : Demux  Outputs=2
  Dregulator : Subsystem
  Limita Uq : Subsystem
  Mux : Mux  Inputs=2
  Qregulator : Subsystem
  Udq : Outport
  wires:
  Idqref/1 -> Demux1/1
  Mux/1 -> Udq/1
  Idqdej/1 -> Demux/1
  Limita Uq/1(Uq_lim) -> Qregulator/3(Uqlim), Mux/2
  Dregulator/1(Ud*(-1:1)) -> Mux/1, Limita Uq/1(Ud)
  Demux1/1 -> Dregulator/1(Id*)
  Demux/1 -> Dregulator/2(Iddej)
  Demux1/2 -> Qregulator/2(Iq*)
  Demux/2 -> Qregulator/1(Iqdej)
  Qregulator/1(Uq*(-1:1)) -> Limita Uq/2(Uq)

== system Model_IPS7/Regulacija2/Transformacije ==
  kot : Inport
  I123 : Inport  Port=2
  Udq : Inport  Port=3
  Clarke : Subsystem
  Inverzni Clarke : Subsystem
  Inverzni Park : Subsystem
  Park : Subsystem
  Idq : Outport
  U123 : Outport  Port=2
  wires:
  Inverzni Clarke/1(U_123) -> U123/1
  Park/1(I_dq) -> Idq/1
  kot/1 -> Inverzni Park/1(kot), Park/2(kot)
  Clarke/1(I_ab) -> Park/1(I_ab)
  Inverzni Park/1(U_ab) -> Inverzni Clarke/1(U_ab)
  Udq/1 -> Inverzni Park/2(U_dq)
  I123/1 -> Clarke/1(I_123)

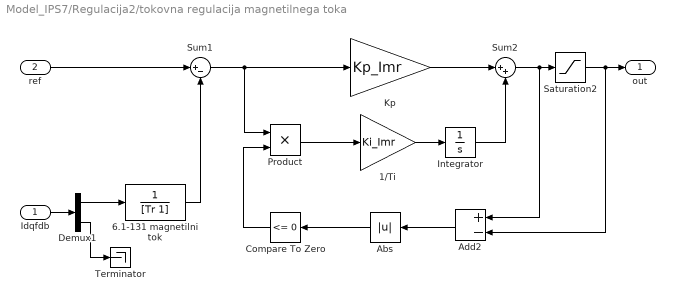
== system Model_IPS7/Regulacija2/tokovna regulacija magnetilnega toka ==
  Idqfdb : Inport
  ref : Inport  Port=2
  1/Ti : Gain  Gain=Ki_Imr  SaturateOnIntegerOverflow=on  OutDataTypeStr=Inherit: Same as input  ParamDataTypeStr=Inherit: Same as input
  6.1-131 magnetilni tok : TransferFcn  Denominator=[Tr 1]
  Abs : Abs
  Add2 : Sum  Inputs=+-
  Compare To Zero : simulink/Logic and Bit Operations/Compare To Zero  relop=<=  OutDataTypeStr=boolean
  Demux1 : Demux  Outputs=2
  Integrator : Integrator
  Kp : Gain  Gain=Kp_Imr  SaturateOnIntegerOverflow=on  OutDataTypeStr=Inherit: Same as input  ParamDataTypeStr=Inherit: Same as input
  Product : Product
  Saturation2 : Saturate  UpperLimit=Ismax  LowerLimit=-Ismax
  Sum1 : Sum  Inputs=|+-
  Sum2 : Sum  Inputs=|++
  Terminator : Terminator
  out : Outport
  wires:
  Product/1 -> 1/Ti/1
  Compare To Zero/1 -> Product/2
  Abs/1 -> Compare To Zero/1
  Add2/1 -> Abs/1
  Integrator/1 -> Sum2/2
  ref/1 -> Sum1/1
  Sum1/1 -> Kp/1, Product/1
  1/Ti/1 -> Integrator/1
  Kp/1 -> Sum2/1
  Demux1/1 -> 6.1-131 magnetilni tok/1
  6.1-131 magnetilni tok/1 -> Sum1/2
  Idqfdb/1 -> Demux1/1
  Sum2/1 -> Add2/1, Saturation2/1
  Saturation2/1 -> Add2/2, out/1
  Demux1/2 -> Terminator/1

== system Model_IPS7/TechniqueB1/Const c ==
  Id : Inport
  6.1-1 : TransferFcn  Numerator=[-Tr*Lm^2/Lr 0]  Denominator=[Tr 1]
  Manual Switch : ManualSwitch
  Scope : Scope  NumInputPorts=2
  Transfer Fcn : TransferFcn  Denominator=[filtkonst 1]
  c : Outport
  wires:
  Id/1 -> 6.1-1/1
  Transfer Fcn/1 -> Scope/2, Manual Switch/1
  Manual Switch/1 -> c/1
  6.1-1/1 -> Scope/1, Manual Switch/2, Transfer Fcn/1

== system Model_IPS7/Time&random/99% max navora ==
  "\tIdq" : Inport
  Iqmax : Inport  Port=2
  Demux : Demux  Outputs=2
  Gain1 : Gain  Gain=3*pp/2
  Gain2 : Gain  Gain=Lm*Lm/Lr
  Product2 : Product  Inputs=3  RndMeth=Zero
  Step : Step  Time=0.6  After=0.99  SampleTime=0
  Out1 : Outport
  wires:
  "\tIdq"/1 -> Demux/1
  Demux/1 -> Product2/1
  Iqmax/1 -> Product2/2
  Step/1 -> Product2/3
  Gain1/1 -> Gain2/1
  Product2/1 -> Gain1/1
  Gain2/1 -> Out1/1

== system Model_IPS7/Asinhronski stroj1/Clarke/ABC_ab1 ==
  A : Inport
  B : Inport  Port=2
  C : Inport  Port=3
  Gain1 : Gain  Gain=2
  Gain2 : Gain
  Gain24 : Gain  Gain=sqrt(3)/3
  Sum11 : Sum
  Terminator : Terminator
  alfa : Outport
  beta : Outport  Port=2
  wires:
  C/1 -> Terminator/1
  Gain1/1 -> Sum11/2
  B/1 -> Gain1/1
  Gain24/1 -> beta/1
  Gain2/1 -> alfa/1
  Sum11/1 -> Gain24/1
  A/1 -> Sum11/1, Gain2/1

== system Model_IPS7/Asinhronski stroj1/Inverzni Clarke/ab_ABC ==
  alfa : Inport
  beta : Inport  Port=2
  Gain1 : Gain
  Gain2 : Gain  Gain=-0.5
  Gain25 : Gain  Gain=sqrt(3)/2
  Gain3 : Gain  Gain=sqrt(3)/2
  Gain4 : Gain  Gain=0.5
  Sum10 : Sum
  Sum11 : Sum  Inputs=--
  A : Outport
  B : Outport  Port=2
  C : Outport  Port=3
  wires:
  Gain3/1 -> Sum11/2
  beta/1 -> Gain25/1, Gain3/1
  Gain4/1 -> Sum11/1
  Gain25/1 -> Sum10/2
  Gain2/1 -> Sum10/1
  alfa/1 -> Gain1/1, Gain2/1, Gain4/1
  Gain1/1 -> A/1
  Sum10/1 -> B/1
  Sum11/1 -> C/1

== system Model_IPS7/Asinhronski stroj1/Mehanika/eq 2.19 ==
  M : Inport
  Gain1 : Gain  Gain=1/J
  Integrator : Integrator
  wr : Outport
  wires:
  Integrator/1 -> wr/1
  M/1 -> Gain1/1
  Gain1/1 -> Integrator/1

== system Model_IPS7/Asinhronski stroj1/napetostni dq model/eq 5.35 ==
  Imr : Inport
  Isq : Inport  Port=2
  Gain : Gain  Gain=3*pp/2
  Gain2 : Gain  Gain=Lm*Lm/Lr
  Product : Product  RndMeth=Zero
  Mel : Outport
  wires:
  Gain/1 -> Gain2/1
  Gain2/1 -> Mel/1
  Product/1 -> Gain/1
  Isq/1 -> Product/2
  Imr/1 -> Product/1

== system Model_IPS7/Asinhronski stroj1/napetostni dq model/eq 5.39 ==
  Isd : Inport
  Gain : Gain  Gain=1/Tr
  Integrator : Integrator  InitialCondition=1e-3
  Sum : Sum  Inputs=|+-
  Imr : Outport
  dImr/dt : Outport  Port=2
  wires:
  Gain/1 -> dImr/dt/1, Integrator/1
  Sum/1 -> Gain/1
  Integrator/1 -> Sum/2, Imr/1
  Isd/1 -> Sum/1

== system Model_IPS7/Asinhronski stroj1/napetostni dq model/eq 5.40 ==
  Imr : Inport
  Isq : Inport  Port=2
  wr_el : Inport  Port=3
  Divide : Product  Inputs=*/
  Gain2 : Gain  Gain=Tr
  Saturation : Saturate  UpperLimit=2*pi*50  LowerLimit=-2*pi*50
  Sum : Sum  Inputs=|++
  wmr : Outport
  wires:
  Saturation/1 -> Sum/1
  Sum/1 -> wmr/1
  wr_el/1 -> Sum/2
  Divide/1 -> Saturation/1  "ws"
  Gain2/1 -> Divide/2
  Imr/1 -> Gain2/1
  Isq/1 -> Divide/1

== system Model_IPS7/Asinhronski stroj1/napetostni dq model/eq 5.46 ==
  Usd : Inport
  dImr/dt : Inport  Port=2
  Isq : Inport  Port=3
  wmr : Inport  Port=4
  Gain : Gain  Gain=1/(sigma*Ls)
  Gain1 : Gain  Gain=Rs
  Gain2 : Gain  Gain=(1-sigma)*Ls
  Gain3 : Gain  Gain=sigma*Ls
  Integrator : Integrator
  Product : Product  RndMeth=Zero
  Sum : Sum  Inputs=+--+
  Isd : Outport
  wires:
  Gain3/1 -> Sum/4
  Product/1 -> Gain3/1
  Isq/1 -> Product/1
  wmr/1 -> Product/2
  Gain2/1 -> Sum/3
  dImr/dt/1 -> Gain2/1
  Gain1/1 -> Sum/2
  Usd/1 -> Sum/1
  Sum/1 -> Gain/1
  Gain/1 -> Integrator/1
  Integrator/1 -> Gain1/1, Isd/1

== system Model_IPS7/Asinhronski stroj1/napetostni dq model/eq 5.47 ==
  Usq : Inport
  Imr : Inport  Port=2
  Isd : Inport  Port=3
  wmr : Inport  Port=4
  Gain : Gain  Gain=1/(sigma*Ls)
  Gain1 : Gain  Gain=Rs
  Gain2 : Gain  Gain=(1-sigma)*Ls
  Gain3 : Gain  Gain=sigma*Ls
  Integrator : Integrator
  Product : Product  RndMeth=Zero
  Product1 : Product  RndMeth=Zero
  Sum : Sum  Inputs=+---
  Isq : Outport
  wires:
  Gain3/1 -> Sum/4
  Product1/1 -> Gain3/1
  Isd/1 -> Product1/2
  Gain2/1 -> Sum/3
  Product/1 -> Gain2/1
  wmr/1 -> Product1/1, Product/2
  Imr/1 -> Product/1
  Gain1/1 -> Sum/2
  Usq/1 -> Sum/1
  Sum/1 -> Gain/1
  Gain/1 -> Integrator/1
  Integrator/1 -> Gain1/1, Isq/1

== system Model_IPS7/Asinhronski stroj2/Clarke/ABC_ab1 ==
  A : Inport
  B : Inport  Port=2
  C : Inport  Port=3
  Gain1 : Gain  Gain=2
  Gain2 : Gain
  Gain24 : Gain  Gain=sqrt(3)/3
  Sum11 : Sum
  Terminator : Terminator
  alfa : Outport
  beta : Outport  Port=2
  wires:
  C/1 -> Terminator/1
  Gain1/1 -> Sum11/2
  B/1 -> Gain1/1
  Gain24/1 -> beta/1
  Gain2/1 -> alfa/1
  Sum11/1 -> Gain24/1
  A/1 -> Sum11/1, Gain2/1

== system Model_IPS7/Asinhronski stroj2/Inverzni Clarke/ab_ABC ==
  alfa : Inport
  beta : Inport  Port=2
  Gain1 : Gain
  Gain2 : Gain  Gain=-0.5
  Gain25 : Gain  Gain=sqrt(3)/2
  Gain3 : Gain  Gain=sqrt(3)/2
  Gain4 : Gain  Gain=0.5
  Sum10 : Sum
  Sum11 : Sum  Inputs=--
  A : Outport
  B : Outport  Port=2
  C : Outport  Port=3
  wires:
  Gain3/1 -> Sum11/2
  beta/1 -> Gain25/1, Gain3/1
  Gain4/1 -> Sum11/1
  Gain25/1 -> Sum10/2
  Gain2/1 -> Sum10/1
  alfa/1 -> Gain1/1, Gain2/1, Gain4/1
  Gain1/1 -> A/1
  Sum10/1 -> B/1
  Sum11/1 -> C/1

== system Model_IPS7/Asinhronski stroj2/Mehanika/eq 2.19 ==
  M : Inport
  Gain1 : Gain  Gain=1/J
  Integrator : Integrator
  wr : Outport
  wires:
  Integrator/1 -> wr/1
  M/1 -> Gain1/1
  Gain1/1 -> Integrator/1

== system Model_IPS7/Asinhronski stroj2/napetostni dq model/eq 5.35 ==
  Imr : Inport
  Isq : Inport  Port=2
  Gain : Gain  Gain=3*pp/2
  Gain2 : Gain  Gain=Lm*Lm/Lr
  Product : Product  RndMeth=Zero
  Mel : Outport
  wires:
  Gain/1 -> Gain2/1
  Gain2/1 -> Mel/1
  Product/1 -> Gain/1
  Isq/1 -> Product/2
  Imr/1 -> Product/1

== system Model_IPS7/Asinhronski stroj2/napetostni dq model/eq 5.39 ==
  Isd : Inport
  Gain : Gain  Gain=1/Tr
  Integrator : Integrator  InitialCondition=1e-3
  Sum : Sum  Inputs=|+-
  Imr : Outport
  dImr/dt : Outport  Port=2
  wires:
  Gain/1 -> dImr/dt/1, Integrator/1
  Sum/1 -> Gain/1
  Integrator/1 -> Sum/2, Imr/1
  Isd/1 -> Sum/1

== system Model_IPS7/Asinhronski stroj2/napetostni dq model/eq 5.40 ==
  Imr : Inport
  Isq : Inport  Port=2
  wr_el : Inport  Port=3
  Divide : Product  Inputs=*/
  Gain2 : Gain  Gain=Tr
  Saturation : Saturate  UpperLimit=2*pi*50  LowerLimit=-2*pi*50
  Sum : Sum  Inputs=|++
  wmr : Outport
  wires:
  Saturation/1 -> Sum/1
  Sum/1 -> wmr/1
  wr_el/1 -> Sum/2
  Divide/1 -> Saturation/1  "ws"
  Gain2/1 -> Divide/2
  Imr/1 -> Gain2/1
  Isq/1 -> Divide/1

== system Model_IPS7/Asinhronski stroj2/napetostni dq model/eq 5.46 ==
  Usd : Inport
  dImr/dt : Inport  Port=2
  Isq : Inport  Port=3
  wmr : Inport  Port=4
  Gain : Gain  Gain=1/(sigma*Ls)
  Gain1 : Gain  Gain=Rs
  Gain2 : Gain  Gain=(1-sigma)*Ls
  Gain3 : Gain  Gain=sigma*Ls
  Integrator : Integrator
  Product : Product  RndMeth=Zero
  Sum : Sum  Inputs=+--+
  Isd : Outport
  wires:
  Gain3/1 -> Sum/4
  Product/1 -> Gain3/1
  Isq/1 -> Product/1
  wmr/1 -> Product/2
  Gain2/1 -> Sum/3
  dImr/dt/1 -> Gain2/1
  Gain1/1 -> Sum/2
  Usd/1 -> Sum/1
  Sum/1 -> Gain/1
  Gain/1 -> Integrator/1
  Integrator/1 -> Gain1/1, Isd/1

== system Model_IPS7/Asinhronski stroj2/napetostni dq model/eq 5.47 ==
  Usq : Inport
  Imr : Inport  Port=2
  Isd : Inport  Port=3
  wmr : Inport  Port=4
  Gain : Gain  Gain=1/(sigma*Ls)
  Gain1 : Gain  Gain=Rs
  Gain2 : Gain  Gain=(1-sigma)*Ls
  Gain3 : Gain  Gain=sigma*Ls
  Integrator : Integrator
  Product : Product  RndMeth=Zero
  Product1 : Product  RndMeth=Zero
  Sum : Sum  Inputs=+---
  Isq : Outport
  wires:
  Gain3/1 -> Sum/4
  Product1/1 -> Gain3/1
  Isd/1 -> Product1/2
  Gain2/1 -> Sum/3
  Product/1 -> Gain2/1
  wmr/1 -> Product1/1, Product/2
  Imr/1 -> Product/1
  Gain1/1 -> Sum/2
  Usq/1 -> Sum/1
  Sum/1 -> Gain/1
  Gain/1 -> Integrator/1
  Integrator/1 -> Gain1/1, Isq/1

== system Model_IPS7/Regulacija1/Regulacija navora/Limita q toka ==
  Iddej : Inport
  wfdb : Inport  Port=2
  Iq* : Inport  Port=3
  0 : Constant  Value=0
  Saturation napetost : simulink/Discontinuities/Saturation Dynamic  OutMin=[]  OutMax=[]  OutDataTypeStr=Inherit: Same as second input  OutDataType=fixdt(1, 16)  OutScaling=2^-10  DoSatur=off
  Saturation presek : simulink/Discontinuities/Saturation Dynamic  OutMin=[]  OutMax=[]  OutDataTypeStr=Inherit: Same as second input  OutDataType=fixdt(1, 16)  OutScaling=2^-10  DoSatur=off
  Saturation tok : simulink/Discontinuities/Saturation Dynamic  OutMin=[]  OutMax=[]  OutDataTypeStr=Inherit: Same as second input  OutDataType=fixdt(1, 16)  OutScaling=2^-10  DoSatur=off
  napetostna limita : Subsystem
  tokovna : Subsystem
  Iqmaxlim : Outport
  Iq*_lim : Outport  Port=2
  wires:
  wfdb/1 -> napetostna limita/2(w)
  napetostna limita/1(high) -> Saturation napetost/1, Saturation presek/1
  Iddej/1 -> napetostna limita/1(Iddej), tokovna/1(Id)
  tokovna/2(low) -> Saturation tok/3
  tokovna/1(high) -> Saturation tok/1, Saturation presek/2
  Saturation presek/1 -> Iqmaxlim/1
  napetostna limita/2(low) -> Saturation napetost/3
  Saturation tok/1 -> Saturation napetost/2
  Iq*/1 -> Saturation tok/2
  Saturation napetost/1 -> Iq*_lim/1
  0/1 -> Saturation presek/3

== system Model_IPS7/Regulacija1/Tok regulator/Dregulator ==
  Id* : Inport
  Iddej : Inport  Port=2
  1/Ti : Gain  Gain=Ki_tok  SaturateOnIntegerOverflow=on  OutDataTypeStr=Inherit: Same as input  ParamDataTypeStr=Inherit: Same as input
  Abs : Abs  ZeroCross=off
  Add2 : Sum  Inputs=+-
  Compare To Zero : simulink/Logic and Bit Operations/Compare To Zero  relop=<=  OutDataTypeStr=boolean  ZeroCross=off
  Integrator : Integrator
  Kp : Gain  Gain=Kp_tok  SaturateOnIntegerOverflow=on  OutDataTypeStr=Inherit: Same as input  ParamDataTypeStr=Inherit: Same as input
  Product : Product
  Saturation : Saturate  UpperLimit=0.990  LowerLimit=-0.990  ZeroCross=off
  Sum1 : Sum  Inputs=|+-
  Sum2 : Sum  Inputs=|++
  Ud*(-1:1) : Outport
  wires:
  Sum1/1 -> Product/1, Kp/1
  Add2/1 -> Abs/1
  Abs/1 -> Compare To Zero/1
  Iddej/1 -> Sum1/2
  1/Ti/1 -> Integrator/1
  Product/1 -> 1/Ti/1
  Kp/1 -> Sum2/1
  Compare To Zero/1 -> Product/2
  Sum2/1 -> Add2/1, Saturation/1
  Integrator/1 -> Sum2/2
  Id*/1 -> Sum1/1
  Saturation/1 -> Add2/2, Ud*(-1:1)/1

== system Model_IPS7/Regulacija1/Tok regulator/Limita Uq ==
  Ud : Inport
  Uq : Inport  Port=2
  Abs : Abs
  Add : Sum  Inputs=+-
  Constant1 : Constant
  Gain : Gain  Gain=-1
  Product3 : Product
  Saturation Dynamic : simulink/Discontinuities/Saturation Dynamic  OutMin=[]  OutMax=[]  OutDataTypeStr=Inherit: Same as second input  OutDataType=fixdt(1, 16)  OutScaling=2^-10  DoSatur=off
  Sqrt : Sqrt  SaturateOnIntegerOverflow=on
  Uq_lim : Outport
  wires:
  Ud/1 -> Product3/1, Product3/2
  Uq/1 -> Saturation Dynamic/2
  Saturation Dynamic/1 -> Uq_lim/1
  Constant1/1 -> Add/1
  Gain/1 -> Saturation Dynamic/3
  Product3/1 -> Add/2
  Add/1 -> Sqrt/1
  Sqrt/1 -> Abs/1
  Abs/1 -> Saturation Dynamic/1, Gain/1

== system Model_IPS7/Regulacija1/Tok regulator/Qregulator ==
  Iqdej : Inport
  Iq* : Inport  Port=2
  Uqlim : Inport  Port=3
  1/Ti1 : Gain  Gain=Ki_tok  SaturateOnIntegerOverflow=on  OutDataTypeStr=Inherit: Same as input  ParamDataTypeStr=Inherit: Same as input
  Abs1 : Abs
  Add1 : Sum  Inputs=+-
  Compare To Zero1 : simulink/Logic and Bit Operations/Compare To Zero  relop=<=  OutDataTypeStr=boolean
  Integrator1 : Integrator
  Kp1 : Gain  Gain=Kp_tok  SaturateOnIntegerOverflow=on  OutDataTypeStr=Inherit: Same as input  ParamDataTypeStr=Inherit: Same as input
  Product1 : Product
  Sum3 : Sum  Inputs=|+-
  Sum4 : Sum  Inputs=|++
  Uq*(-1:1) : Outport
  wires:
  Iq*/1 -> Sum3/1
  Kp1/1 -> Sum4/1
  Integrator1/1 -> Sum4/2
  Sum3/1 -> Kp1/1, Product1/1
  Add1/1 -> Abs1/1
  Compare To Zero1/1 -> Product1/2
  Product1/1 -> 1/Ti1/1
  1/Ti1/1 -> Integrator1/1
  Abs1/1 -> Compare To Zero1/1
  Iqdej/1 -> Sum3/2
  Sum4/1 -> Uq*(-1:1)/1, Add1/1
  Uqlim/1 -> Add1/2

== system Model_IPS7/Regulacija1/Transformacije/Clarke ==
  I_123 : Inport
  ABC_ab1 : Subsystem
  Demux : Demux  Outputs=3
  Mux : Mux  Inputs=2
  I_ab : Outport
  wires:
  Mux/1 -> I_ab/1
  ABC_ab1/2(beta) -> Mux/2
  ABC_ab1/1(alfa) -> Mux/1
  Demux/3 -> ABC_ab1/3(C)
  Demux/2 -> ABC_ab1/2(B)
  Demux/1 -> ABC_ab1/1(A)
  I_123/1 -> Demux/1

== system Model_IPS7/Regulacija1/Transformacije/Inverzni Clarke ==
  U_ab : Inport
  Demux : Demux  Outputs=2
  Mux : Mux  Inputs=3
  ab_ABC : Subsystem
  U_123 : Outport
  wires:
  ab_ABC/3(C) -> Mux/3
  ab_ABC/2(B) -> Mux/2
  ab_ABC/1(A) -> Mux/1
  Demux/2 -> ab_ABC/2(beta)
  Demux/1 -> ab_ABC/1(alfa)
  U_ab/1 -> Demux/1
  Mux/1 -> U_123/1

== system Model_IPS7/Regulacija1/Transformacije/Inverzni Park ==
  kot : Inport
  U_dq : Inport  Port=2
  Demux : Demux  Outputs=2
  Mux : Mux  Inputs=2
  "Sum1 " : Sum  Inputs=+-  SaturateOnIntegerOverflow=on  InputSameDT=on  OutDataTypeStr=Inherit: Same as first input
  Sum2 : Sum  SaturateOnIntegerOverflow=on  InputSameDT=on  OutDataTypeStr=Inherit: Same as first input
  cos : Fcn  Expr=cos(u)
  sin : Fcn  Expr=sin(u)
  x_d*cos : Product  SaturateOnIntegerOverflow=on  RndMeth=Zero  InputSameDT=on  OutDataTypeStr=Inherit: Same as first input
  x_d*sin : Product  SaturateOnIntegerOverflow=on  RndMeth=Zero  InputSameDT=on  OutDataTypeStr=Inherit: Same as first input
  x_q*cos : Product  SaturateOnIntegerOverflow=on  RndMeth=Zero  InputSameDT=on  OutDataTypeStr=Inherit: Same as first input
  "x_q*sin " : Product  SaturateOnIntegerOverflow=on  RndMeth=Zero  InputSameDT=on  OutDataTypeStr=Inherit: Same as first input
  U_ab : Outport
  wires:
  Mux/1 -> U_ab/1
  U_dq/1 -> Demux/1
  Demux/1 -> x_d*sin/1, x_d*cos/1
  Demux/2 -> "x_q*sin "/1, x_q*cos/1
  cos/1 -> x_q*cos/2, x_d*cos/2
  sin/1 -> "x_q*sin "/2, x_d*sin/2
  x_d*cos/1 -> "Sum1 "/1
  "x_q*sin "/1 -> "Sum1 "/2
  x_q*cos/1 -> Sum2/2
  x_d*sin/1 -> Sum2/1
  "Sum1 "/1 -> Mux/1
  Sum2/1 -> Mux/2
  kot/1 -> cos/1, sin/1

== system Model_IPS7/Regulacija1/Transformacije/Park ==
  I_ab : Inport
  kot : Inport  Port=2
  Demux : Demux  Outputs=2
  Mux : Mux  Inputs=2
  "Sum1 " : Sum  SaturateOnIntegerOverflow=on  InputSameDT=on  OutDataTypeStr=Inherit: Same as first input
  Sum2 : Sum  Inputs=-+  SaturateOnIntegerOverflow=on  InputSameDT=on  OutDataTypeStr=Inherit: Same as first input
  cos : Fcn  Expr=cos(u)
  sin : Fcn  Expr=sin(u)
  x_a*cos : Product  SaturateOnIntegerOverflow=on  RndMeth=Zero  InputSameDT=on  OutDataTypeStr=Inherit: Same as first input
  x_a*sin : Product  SaturateOnIntegerOverflow=on  RndMeth=Zero  InputSameDT=on  OutDataTypeStr=Inherit: Same as first input
  x_b*cos : Product  SaturateOnIntegerOverflow=on  RndMeth=Zero  InputSameDT=on  OutDataTypeStr=Inherit: Same as first input
  "x_b*sin " : Product  SaturateOnIntegerOverflow=on  RndMeth=Zero  InputSameDT=on  OutDataTypeStr=Inherit: Same as first input
  I_dq : Outport
  wires:
  Mux/1 -> I_dq/1
  I_ab/1 -> Demux/1
  Demux/1 -> x_a*sin/1, x_a*cos/1
  Demux/2 -> "x_b*sin "/1, x_b*cos/1
  cos/1 -> x_b*cos/2, x_a*cos/2
  sin/1 -> "x_b*sin "/2, x_a*sin/2
  x_a*cos/1 -> "Sum1 "/1
  "x_b*sin "/1 -> "Sum1 "/2
  x_b*cos/1 -> Sum2/2
  x_a*sin/1 -> Sum2/1
  "Sum1 "/1 -> Mux/1
  Sum2/1 -> Mux/2
  kot/1 -> cos/1, sin/1

== system Model_IPS7/Regulacija2/Regulacija navora/Limita q toka ==
  Iddej : Inport
  wfdb : Inport  Port=2
  Iq* : Inport  Port=3
  0 : Constant  Value=0
  Saturation napetost : simulink/Discontinuities/Saturation Dynamic  OutMin=[]  OutMax=[]  OutDataTypeStr=Inherit: Same as second input  OutDataType=fixdt(1, 16)  OutScaling=2^-10  DoSatur=off
  Saturation presek : simulink/Discontinuities/Saturation Dynamic  OutMin=[]  OutMax=[]  OutDataTypeStr=Inherit: Same as second input  OutDataType=fixdt(1, 16)  OutScaling=2^-10  DoSatur=off
  Saturation tok : simulink/Discontinuities/Saturation Dynamic  OutMin=[]  OutMax=[]  OutDataTypeStr=Inherit: Same as second input  OutDataType=fixdt(1, 16)  OutScaling=2^-10  DoSatur=off
  napetostna limita : Subsystem
  tokovna : Subsystem
  Iqmaxlim : Outport
  Iq*_lim : Outport  Port=2
  wires:
  wfdb/1 -> napetostna limita/2(w)
  napetostna limita/1(high) -> Saturation napetost/1, Saturation presek/1
  Iddej/1 -> napetostna limita/1(Iddej), tokovna/1(Id)
  tokovna/2(low) -> Saturation tok/3
  tokovna/1(high) -> Saturation tok/1, Saturation presek/2
  Saturation presek/1 -> Iqmaxlim/1
  napetostna limita/2(low) -> Saturation napetost/3
  Saturation tok/1 -> Saturation napetost/2
  Iq*/1 -> Saturation tok/2
  Saturation napetost/1 -> Iq*_lim/1
  0/1 -> Saturation presek/3

== system Model_IPS7/Regulacija2/Tok regulator/Dregulator ==
  Id* : Inport
  Iddej : Inport  Port=2
  1/Ti : Gain  Gain=Ki_tok  SaturateOnIntegerOverflow=on  OutDataTypeStr=Inherit: Same as input  ParamDataTypeStr=Inherit: Same as input
  Abs : Abs  ZeroCross=off
  Add2 : Sum  Inputs=+-
  Compare To Zero : simulink/Logic and Bit Operations/Compare To Zero  relop=<=  OutDataTypeStr=boolean  ZeroCross=off
  Integrator : Integrator
  Kp : Gain  Gain=Kp_tok  SaturateOnIntegerOverflow=on  OutDataTypeStr=Inherit: Same as input  ParamDataTypeStr=Inherit: Same as input
  Product : Product
  Saturation : Saturate  UpperLimit=0.990  LowerLimit=-0.990  ZeroCross=off
  Sum1 : Sum  Inputs=|+-
  Sum2 : Sum  Inputs=|++
  Ud*(-1:1) : Outport
  wires:
  Sum1/1 -> Product/1, Kp/1
  Add2/1 -> Abs/1
  Abs/1 -> Compare To Zero/1
  Iddej/1 -> Sum1/2
  1/Ti/1 -> Integrator/1
  Product/1 -> 1/Ti/1
  Kp/1 -> Sum2/1
  Compare To Zero/1 -> Product/2
  Sum2/1 -> Add2/1, Saturation/1
  Integrator/1 -> Sum2/2
  Id*/1 -> Sum1/1
  Saturation/1 -> Add2/2, Ud*(-1:1)/1

== system Model_IPS7/Regulacija2/Tok regulator/Limita Uq ==
  Ud : Inport
  Uq : Inport  Port=2
  Abs : Abs
  Add : Sum  Inputs=+-
  Constant1 : Constant
  Gain : Gain  Gain=-1
  Product3 : Product
  Saturation Dynamic : simulink/Discontinuities/Saturation Dynamic  OutMin=[]  OutMax=[]  OutDataTypeStr=Inherit: Same as second input  OutDataType=fixdt(1, 16)  OutScaling=2^-10  DoSatur=off
  Sqrt : Sqrt  SaturateOnIntegerOverflow=on
  Uq_lim : Outport
  wires:
  Ud/1 -> Product3/1, Product3/2
  Uq/1 -> Saturation Dynamic/2
  Saturation Dynamic/1 -> Uq_lim/1
  Constant1/1 -> Add/1
  Gain/1 -> Saturation Dynamic/3
  Product3/1 -> Add/2
  Add/1 -> Sqrt/1
  Sqrt/1 -> Abs/1
  Abs/1 -> Saturation Dynamic/1, Gain/1

== system Model_IPS7/Regulacija2/Tok regulator/Qregulator ==
  Iqdej : Inport
  Iq* : Inport  Port=2
  Uqlim : Inport  Port=3
  1/Ti1 : Gain  Gain=Ki_tok  SaturateOnIntegerOverflow=on  OutDataTypeStr=Inherit: Same as input  ParamDataTypeStr=Inherit: Same as input
  Abs1 : Abs
  Add1 : Sum  Inputs=+-
  Compare To Zero1 : simulink/Logic and Bit Operations/Compare To Zero  relop=<=  OutDataTypeStr=boolean
  Integrator1 : Integrator
  Kp1 : Gain  Gain=Kp_tok  SaturateOnIntegerOverflow=on  OutDataTypeStr=Inherit: Same as input  ParamDataTypeStr=Inherit: Same as input
  Product1 : Product
  Sum3 : Sum  Inputs=|+-
  Sum4 : Sum  Inputs=|++
  Uq*(-1:1) : Outport
  wires:
  Iq*/1 -> Sum3/1
  Kp1/1 -> Sum4/1
  Integrator1/1 -> Sum4/2
  Sum3/1 -> Kp1/1, Product1/1
  Add1/1 -> Abs1/1
  Compare To Zero1/1 -> Product1/2
  Product1/1 -> 1/Ti1/1
  1/Ti1/1 -> Integrator1/1
  Abs1/1 -> Compare To Zero1/1
  Iqdej/1 -> Sum3/2
  Sum4/1 -> Uq*(-1:1)/1, Add1/1
  Uqlim/1 -> Add1/2

== system Model_IPS7/Regulacija2/Transformacije/Clarke ==
  I_123 : Inport
  ABC_ab1 : Subsystem
  Demux : Demux  Outputs=3
  Mux : Mux  Inputs=2
  I_ab : Outport
  wires:
  Mux/1 -> I_ab/1
  ABC_ab1/2(beta) -> Mux/2
  ABC_ab1/1(alfa) -> Mux/1
  Demux/3 -> ABC_ab1/3(C)
  Demux/2 -> ABC_ab1/2(B)
  Demux/1 -> ABC_ab1/1(A)
  I_123/1 -> Demux/1

== system Model_IPS7/Regulacija2/Transformacije/Inverzni Clarke ==
  U_ab : Inport
  Demux : Demux  Outputs=2
  Mux : Mux  Inputs=3
  ab_ABC : Subsystem
  U_123 : Outport
  wires:
  ab_ABC/3(C) -> Mux/3
  ab_ABC/2(B) -> Mux/2
  ab_ABC/1(A) -> Mux/1
  Demux/2 -> ab_ABC/2(beta)
  Demux/1 -> ab_ABC/1(alfa)
  U_ab/1 -> Demux/1
  Mux/1 -> U_123/1
